simulink subsystem "ControlSubsystem_with_IO"  (R2023a)
settings: Solver=VariableStepAuto  StartTime=0.0  StopTime=10.0  RelTol=1e-3
libraries: eeGeneralControl x1
settings Model: Creator=thesa  LastModifiedBy=thesa

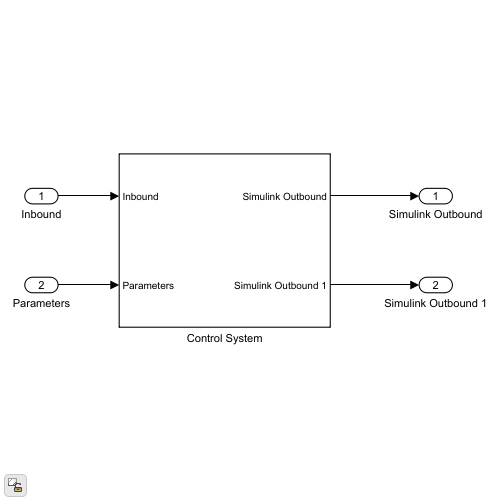
[thumbnail: Simulink's stored preview of the top-level diagram]
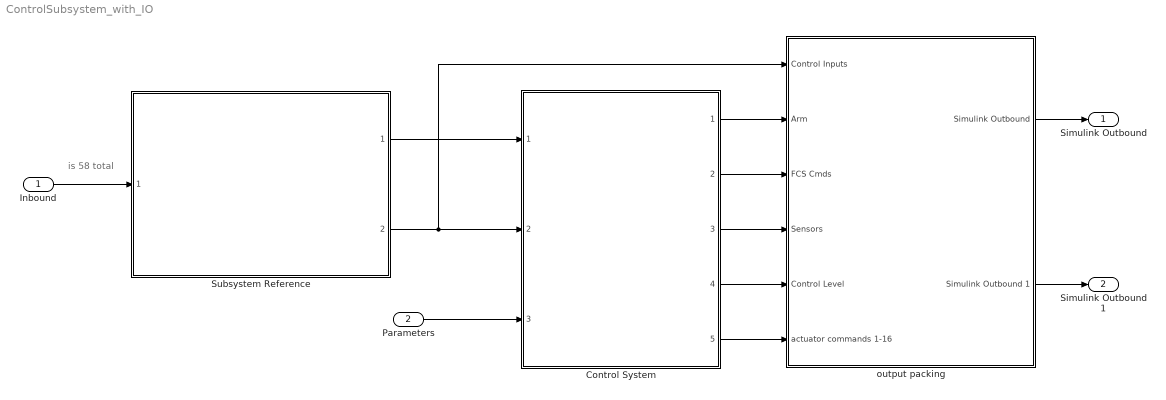
== system ControlSubsystem_with_IO ==
  note: is 58 total
  Inbound : Inport
  Parameters : Inport  Port=2
  Control System : Subsystem  ReferencedSubsystem=Control_System
  Subsystem Reference : Subsystem  ReferencedSubsystem=sm_inbound_interpreter
  output packing : Subsystem
  Simulink Outbound : Outport
  Simulink Outbound 1 : Outport  Port=2
  wires:
  Parameters/1 -> Control System/3
  Inbound/1 -> Subsystem Reference/1
  Subsystem Reference/1 -> Control System/1
  Subsystem Reference/2 -> Control System/2, output packing/1(Control Inputs)
  Control System/1 -> output packing/2(Arm)
  Control System/2 -> output packing/3(FCS Cmds)
  Control System/3 -> output packing/4(Sensors)
  Control System/4 -> output packing/5(Control Level)
  Control System/5 -> output packing/6(actuator commands 1-16)
  output packing/1(Simulink Outbound) -> Simulink Outbound/1
  output packing/2(Simulink Outbound 1) -> Simulink Outbound 1/1

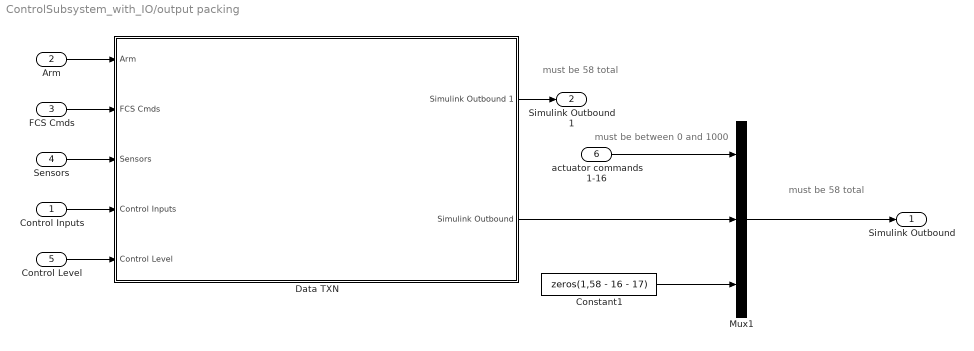
== system ControlSubsystem_with_IO/output packing ==
  note: must be between 0 and 1000
  note: must be 58 total
  note: must be 58 total
  Control Inputs : Inport
  Arm : Inport  Port=2
  FCS Cmds : Inport  Port=3
  Sensors : Inport  Port=4
  Control Level : Inport  Port=5
  actuator commands 1-16 : Inport  Port=6
  Constant1 : Constant  Value=zeros(1,58 - 16 - 17)
  Data TXN : Subsystem
  Mux1 : Mux  Inputs=3
  Simulink Outbound : Outport
  Simulink Outbound 1 : Outport  Port=2
  wires:
  Arm/1 -> Data TXN/1(Arm)
  Sensors/1 -> Data TXN/3(Sensors)
  actuator commands 1-16/1 -> Mux1/1
  Mux1/1 -> Simulink Outbound/1
  Data TXN/2(Simulink Outbound) -> Mux1/2
  Control Level/1 -> Data TXN/5(Control Level)
  FCS Cmds/1 -> Data TXN/2(FCS Cmds)
  Data TXN/1(Simulink Outbound 1) -> Simulink Outbound 1/1
  Constant1/1 -> Mux1/3
  Control Inputs/1 -> Data TXN/4(Control Inputs)

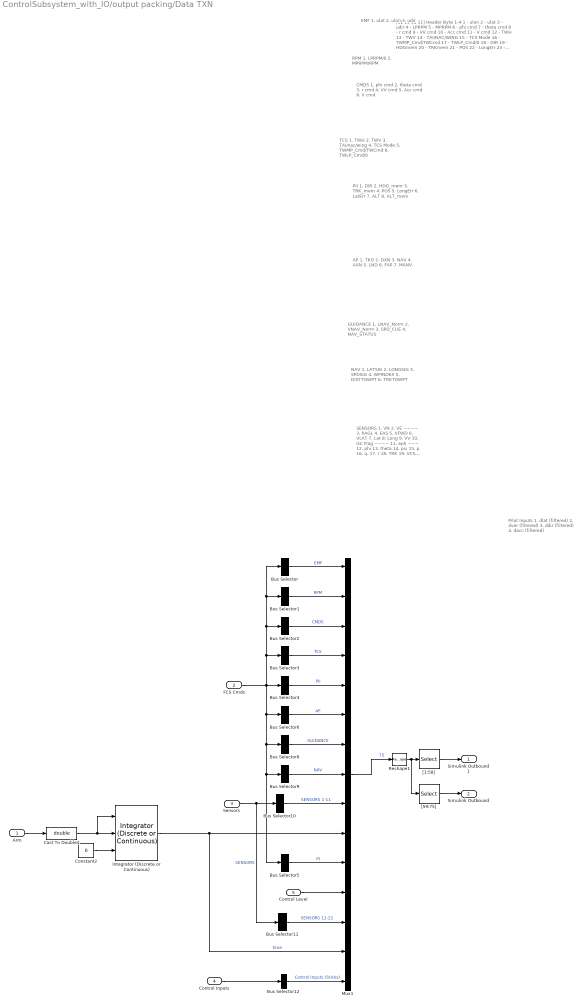
== system ControlSubsystem_with_IO/output packing/Data TXN ==
  note: SENSORS
      | 1. VN
      | 2. VE
      | ~~~~
      | 3. hAGL
      | 4. EAS
      | 5. VFWD
      | 6. VLAT
      | 7. Lat
      | 8. Long
      | 9. VV
      | 10. GC Flag
      | ~~~~
      | 11. eph
      | ~~~
      | 12. phi
      | 13. theta
      | 14. psi
      | 15. p
      | 16. q.
      | 17. r
      | 18. TRK
      | 19. VCS
      | 20. ax
      | 21. ay
      | 22. az
  note: TCS
      | 1. TWH
      | 2. TWV
      | 3. TAI/nac/wing
      | 4. TCS Mode
      | 5. TWMP_Cmd/TWCmd
      | 6. TWLP_Cmd/0
  note: AP
      |
      | 1. TKO
      | 2. DXN
      | 3. NAV
      | 4. AXN
      | 5. LND
      | 6. FAP
      | 7. MANV
  note: Pilot Inputs
      |
      | 1. dlat (filtered)
      | 2. dver (filtered)
      | 3. ddir (filtered)
      | 4. dacc (filtered)
  note: GUIDANCE
      |
      | 1. LNAV_Norm
      | 2. VNAV_Norm
      | 3. SPD_CUE
      | 4. NAV_STATUS
  note: [11 11 11 11] Header Byte 1-4
      | 1 - ulon
      | 2 - ulat
      | 3 - udir
      |
      | 4 - LPRPM
      | 5 - MPRPM
      |
      | 6 - phi cmd
      | 7 - theta cmd
      | 8 - r cmd
      | 9 - VV cmd
      | 10 - Acc cmd
      | 11 - V cmd
      |
      | 12 - TWH
      | 13 - TWV
      | 14 - TAI/NAC/WING
      | 15 - TCS Mode
      | 16 - TWMP_Cmd/TWCmd
      | 17 - TWLP_Cmd/0
      |
      | 18 - DIR
      | 19 - HDGmem
      | 20 - TRKmem
      | 21 - POS
      | 22 - LongErr
      | 23 - LatErr
      | 24 - ALT
      | 25 - ALTmem
      |
      | 26 - TKO
      | 27 - DXN
      | 28 - NAV
      | 29 - AXN
      | 30 - LND
      | 31 - FAP
      | 32 - MANV
      |
      | 33 - LNAV_Norm
      | 34 - VNAV_Norm
      | 35 - SPD_CUE
      | 36 - NAV_STATUS
      |
      | 37 - LATSIG
      | 38 - LONGSIG
      | 39 - SPDSIG
      | 40 - WPINDEX
      | 41 - DISTTOWPT
      | 42 - TRKTOWPT
      |
      | 43 - VN
      | 44 - VE
      | 45 - hAGL
      | 46 - EAS
      | 47 - VFWD
      | 48 - VLAT
      | 49 - Lat
      | 50 - Long
      | 51 - VV
      | 52 - GC Flag
      | 53 - eph
      |
      | 54 - time
      |
      | 55 - dlat
      | 56 - dver
      | 57 - ddir
      | 58 - dacc
      |
      | 59 - Control Level
      |
      | 60 - phi
      | 61 - theta
      | 62 - psi
      | 63 - p
      | 64 - q
      | 65 - r
      | 66 - TRK
      | 67 - VCS
      | 68 - ax
      | 69 - ay
      | 70 - az
      | 71 - time
      | 72 - roll
      | 73 - pitch
      | 74 - yaw
      | 75 - throttle
      | [10 10 10 10] Terminator Byte 284
  note: EMF
      | 1. ulat
      | 2. ulon
      | 3. udir
  note: PII
      |
      | 1. DIR
      | 2. HDG_mem
      | 3. TRK_mem
      | 4. POS
      | 5. LongErr
      | 6. LatErr
      | 7. ALT
      | 8. ALT_mem
  note: RPM
      | 1. LPRPM/0
      | 2. MPRPM/RPM
  note: CMDS
      | 1. phi cmd
      | 2. theta cmd
      | 3. r cmd
      | 4. VV cmd
      | 5. Acc cmd
      | 6. V cmd
  note: NAV
      |
      | 1. LATSIG
      | 2. LONGSIG
      | 3. SPDSIG
      | 4. WPINDEX
      | 5. DISTTOWPT
      | 6. TRKTOWPT
  Arm : Inport
  FCS Cmds : Inport  Port=2
  Sensors : Inport  Port=3
  Control Inputs : Inport  Port=4
  Control Level : Inport  Port=5
  Bus Selector : BusSelector  OutputSignals=EMF.ulat,EMF.ulon,EMF.udir  OutputAsBus=on
  Bus Selector1 : BusSelector  OutputSignals=RPM.LPRPM,RPM.MPRPM  OutputAsBus=on
  Bus Selector10 : BusSelector  OutputSignals=VN,VE,Alt (m),EAS,VFWD (m/s),VLAT (m/s),Lat (deg),Long (deg),VV (m/s),GndContact,eph  OutputAsBus=on
  Bus Selector11 : BusSelector  OutputSignals=phi (rad),theta (rad),HDG (rad),p (rad/s),q (rad/s),r (rad/s),TRK (rad),VCS (kt),ax (m/s2),ay (m/s2),az (m/s2)  OutputAsBus=on
  Bus Selector12 : BusSelector  OutputSignals=Roll,Pitch,Yaw,Throttle  OutputAsBus=on
  Bus Selector2 : BusSelector  OutputSignals=PII.phiCmd,TCS.PitchCmd,PII.rCmd,PII.VV Cmd,PII.Acc Cmd,PII.V Cmd  OutputAsBus=on
  Bus Selector3 : BusSelector  OutputSignals=TCS.TWH,TCS.TWV,TCS.WingCmd,TCS.TCS_Mode,TCS.TWMP_Cmd,TCS.TWLP_Cmd  OutputAsBus=on
  Bus Selector4 : BusSelector  OutputSignals=PII.DIR,PII.HDGmem,PII.TRKmem,PII.POS,PII.LongErr,PII.LatErr,PII.ALT,PII.ALTmem  OutputAsBus=on
  Bus Selector5 : BusSelector  OutputSignals=PII.dlat,PII.dver,PII.ddir,PII.dacc  OutputAsBus=on
  Bus Selector6 : BusSelector  OutputSignals=AP.TKO,AP.DXN,AP.NAV,AP.AXN,AP.LDG,AP.FAP,AP.MANV  OutputAsBus=on
  Bus Selector8 : BusSelector  OutputSignals=GUIDANCE.LNAV_NORM,GUIDANCE.VNAV_NORM,GUIDANCE.SPD_CUE,NAV.NAVSTATUS  OutputAsBus=on
  Bus Selector9 : BusSelector  OutputSignals=NAV.LATSIG,NAV.LONGSIG,NAV.SPDSIG,NAV.WPINDEX,NAV.DistToTarget,NAV.TRK_target  OutputAsBus=on
  Cast To Double4 : DataTypeConversion  OutDataTypeStr=double  SaturateOnIntegerOverflow=off  RndMeth=Floor
  Constant2 : Constant  Value=0
  Integrator (Discrete or Continuous) : eeGeneralControl/Integrator (Discrete or Continuous)  LabelModeActiveChoice=Discrete  ExternalReset=either  LimitType=Anti-windup  B=inf  A=-inf  Ts=-1
  Mux1 : Mux  Inputs=15
  Reshape1 : Reshape
  "[1:58]" : Selector  InputPortWidth=75  IndexOptions=Index vector (dialog)  Indices=[1:58]  OutputSizes=1
  "[59:75]" : Selector  InputPortWidth=75  IndexOptions=Index vector (dialog)  Indices=[59:75]  OutputSizes=1
  Simulink Outbound 1 : Outport
  Simulink Outbound : Outport  Port=2
  wires:
  Bus Selector12/1 -> Mux1/15  "Control Inputs (Sticks)"
  Control Inputs/1 -> Bus Selector12/1
  Bus Selector11/1 -> Mux1/13  "SENSORS 12-22"
  Sensors/1 -> Bus Selector10/1, Bus Selector11/1  "SENSORS"
  "[59:75]"/1 -> Simulink Outbound/1
  "[1:58]"/1 -> Simulink Outbound 1/1
  Reshape1/1 -> "[1:58]"/1, "[59:75]"/1
  Bus Selector9/1 -> Mux1/8  "NAV"
  Bus Selector8/1 -> Mux1/7  "GUIDANCE"
  Bus Selector/1 -> Mux1/1  "EMF"
  Control Level/1 -> Mux1/12
  FCS Cmds/1 -> Bus Selector4/1, Bus Selector3/1, Bus Selector1/1, Bus Selector/1, Bus Selector2/1, Bus Selector5/1, Bus Selector9/1, Bus Selector8/1, Bus Selector6/1
  Bus Selector6/1 -> Mux1/6  "AP"
  Bus Selector1/1 -> Mux1/2  "RPM"
  Arm/1 -> Cast To Double4/1
  Bus Selector10/1 -> Mux1/9  "SENSORS 1-11"
  Mux1/1 -> Reshape1/1  "75"
  Integrator (Discrete or Continuous)/1 -> Mux1/10, Mux1/14  "time"
  Bus Selector3/1 -> Mux1/4  "TCS"
  Bus Selector4/1 -> Mux1/5  "PII"
  Bus Selector2/1 -> Mux1/3  "CMDS"
  Constant2/1 -> Integrator (Discrete or Continuous)/3
  Cast To Double4/1 -> Integrator (Discrete or Continuous)/2, Integrator (Discrete or Continuous)/1
  Bus Selector5/1 -> Mux1/11  "PI"
